simulink model "NeuronalNetwork"  (R2019b)
settings: Solver=VariableStepAuto  StartTime=0.0  StopTime=10.0  RelTol=1e-3
libraries: neural x1006
(part 1 of 11)
settings Model: Creator=Laura  LastModifiedBy=Laura

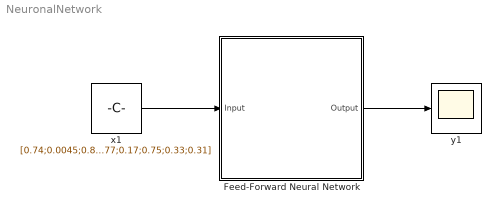
== system NeuronalNetwork ==
  Feed-Forward Neural Network : Subsystem
      mask help: Feed-Forward Neural Network
      mask Display: e = 0.06;c1 = [120 150 230]/255;c2 = ([120 150 230]+0)/383;c3 = ([120 150 230]+128)/383;patch([0 1 1 0],[0 0 1 1],c1);patch([0 1 1 1-e 1-e 0+e],[0 0 1 1-e 0+e 0+e],c2);patch([0 0 1 1-e 0+e 0+e],[0 1 1 1-e 1-e 0+e],c3);plot([0 1 1 0 0],[0 0 1 1 0]);fprintf('NNET');port_label('input',1,' Input');port_label('output',1,'Output ');
  x1 : Constant  Value=[0.74;0.0045;0.85;0.7;0.56;0.34;0.33;0.077;0.46;0.66;0.57;0.4;0.93;0.36;0.95;0.03;0.44;0.7;0.7;0.51;0.61;0.75;0.8;0.34;0.56;0.86;0.59;0.51;0.85;0.68;0.11;0.5;0.019;0.44;0.91;0.045;0.95;0.18;0.37;0.21;0.096;0.43;0.28;0.1;0.5;0.24;0.35;0.56;0.55;0.42;0.39;0.38;0.28;0.18;0.13;0.016;0.75;0.5;0.72;0.76;0.27;0.19;0.064;0.43;0.7;0.98;0.55;0.044;0.58;0.28;0.54;0.44;0.12;0.38;0.76;0.92;0.69;0.97;0.13;0.65;0.39;0.56;0.2;0.39;0.34;0.36;0.37;0.12;0.5;0.82;0.34;0.5;0.12;0.58;0.52;0.36;0.86;0.34;0.46;0.24;0.77;0.27;0.53;0.53;0.87;0.94;0.049;0.98;0.63;0.073;0.21;0.36;0.43;0.76;0.92;0.63;0.96;0.76;0.53;0.85;0.82;0.13;0.76;0.62;0.4;0.84;0.038;0.096;0.95;0.4;0.53;0.9;0.34;0.66;0.73;0.22;0.56;0.46;0.61;0.54;0.52;0.29;0.88;0.94;0.81;0.97;0.52;0.11;0.65;0.19;0.86;0.94;0.1;0.3;0.8;0.44;0.49;0.03;0.57;0.57;0.74;0.077;0.79;0.19;0.53;0.92;0.99;0.98;0.3;0.75;0.21;0.86;0.66;0.1;0.58;0.96;0.84;0.75;0.7;0.25;0.04;0.46;0.12;0.16;0.42;0.67;0.97;0.28;0.53;0.93;0.17;0.79;0.1;0.88;0.52;0.97;0.76;0.72;0.0026;0.21;0.26;0.08;0.74;0.82;0.34;0.14;0.67;0.83;0.67;0.14;0.38;0.68;0.52;0.98;0.27;0.87;0.37;0.14;0.083;0.74;0.37;0.38;0.3;0.29;0.26;0.46;0.99;0.39;0.94;0.17;0.93;0.75;0.86;0.6;0.11;0.46;0.65;0.058;0.021;0.29;0.93;0.51;0.88;0.38;0.88;0.53;0.89;0.1;0.21;0.7;0.36;0.0014;0.38;0.32;0.39;0.18;0.21;0.59;0.59;0.17;0.93;0.056;0.2;0.51;0.76;0.15;0.93;0.42;0.056;0.67;0.28;0.78;0.96;0.69;0.5;0.099;0.29;0.54;0.011;0.28;0.59;0.17;0.17;0.68;0.57;0.55;0.97;0.63;0.32;0.52;0.86;0.99;0.84;0.35;0.75;0.94;0.67;0.48;0.29;0.6;0.34;0.96;0.44;0.96;0.68;0.71;0.96;0.94;0.83;0.16;0.83;0.46;0.3;0.52;0.83;0.54;0.26;0.35;0.19;0.35;0.19;0.84;0.38;0.0095;0.31;0.84;0.28;0.78;0.53;0.15;0.53;0.28;0.71;0.73;0.45;0.18;0.14;0.27;0.64;0.81;0.67;0.29;0.14;0.25;0.69;0.072;0.5;0.99;0.9;0.58;0.77;0.75;0.7;0.68;0.28;0.58;0.62;0.81;0.016;0.21;0.99;0.82;0.63;0.68;0.81;0.28;0.66;0.029;0.54;0.53;0.87;0.19;0.93;0.98;0.33;0.62;0.53;0.46;0.36;0.33;0.083;0.39;0.24;0.49;0.7;0.14;0.83;0.93;0.83;0.48;0.66;0.46;0.42;0.034;0.93;0.043;0.48;0.39;0.53;1;0.9;0.015;0.78;0.49;0.39;0.82;0.87;1;0.2;0.87;0.31;0.41;0.82;0.37;0.43;0.091;0.67;0.73;0.3;0.34;0.73;0.99;0.7;0.09;0.47;0.64;0.53;0.14;0.28;0.99;0.79;0.93;0.35;0.21;0.68;0.36;0.44;0.91;0.83;0.39;0.73;0.29;0.29;0.3;0.025;0.92;0.69;0.23;0.5;0.79;0.38;0.22;0.72;0.77;0.69;0.62;0.76;0.51;0.33;0.0013;0.58;0.17;0.19;0.15;0.51;0.017;0.47;0.046;0.44;0.16;0.57;0.82;0.085;0.23;0.25;0.35;0.41;0.11;0.41;0.68;0.54;0.36;0.66;0.68;0.13;0.44;0.94;0.57;0.58;0.76;0.25;0.69;0.29;0.57;0.63;0.4;0.25;0.94;0.45;0.53;0.63;0.67;0.44;0.17;0.69;0.92;0.37;0.64;0.89;0.48;0.63;0.47;0.11;0.11;0.11;0.45;0.94;0.63;0.93;0.063;0.31;0.95;0.01;0.17;0.76;0.83;0.61;0.52;0.94;0.74;0.7;0.74;0.87;0.96;0.98;0.92;0.28;0.059;0.82;0.18;0.035;0.77;0.54;0.33;0.58;0.85;0.64;0.42;0.55;0.18;0.24;0.21;0.26;0.94;0.64;0.83;0.39;0.17;0.74;0.87;0.36;0.18;1;0.96;0.16;0.93;0.42;0.22;0.14;0.26;0.54;0.082;0.6;0.029;0.45;0.33;0.94;0.3;0.43;0.66;0.38;0.14;0.097;0.31;0.82;0.63;0.21;0.98;0.44;0.84;0.54;0.025;0.0068;0.79;0.45;0.29;0.86;0.66;0.28;0.64;0.26;0.17;0.37;0.54;0.93;0.75;0.15;0.0029;0.13;0.92;0.67;0.11;0.96;0.12;0.49;0.36;0.47;0.059;0.33;0.26;0.25;0.95;0.032;0.91;0.37;0.66;0.95;0.094;0.69;0.41;0.11;0.49;0.46;0.88;0.66;0.28;0.66;0.65;0.9;0.88;0.34;0.43;0.8;0.92;0.87;0.5;0.58;0.92;0.17;0.37;0.26;0.83;0.07;0.28;0.56;0.62;0.41;0.26;0.42;0.38;0.096;0.13;0.61;0.66;0.84;0.5;0.31;0.17;0.049;0.23;0.37;0.57;0.57;0.78;0.59;0.11;0.64;0.072;0.37;0.29;0.74;0.067;0.76;0.24;0.23;0.012;0.13;0.21;0.21;0.91;0.28;0.097;0.78;0.67;0.61;0.34;0.69;0.23;0.31;0.36;0.22;0.68;0.74;0.01;0.36;0.24;0.93;0.76;0.38;0.69;0.7;0.59;0.96;0.78;0.54;0.094;0.89;0.26;0.46;0.33;0.76;0.8;0.8;0.88;0.087;0.67;0.5;0.34;0.59;0.35;0.21;0.26;0.099;0.15;0.32;0.59;0.15;0.063;0.0078;0.77;0.68;0.12;0.72;0.16;0.12;0.68;0.14;0.058;0.13;0.015;0.19;0.071;0.038;0.31;0.52;0.39;1;0.44;0.15;0.78;0.74;0.088;0.47;0.29;0.41;0.43;0.87;0.71;0.014;0.025;0.24;0.6;0.93;0.33;0.44;0.099;0.72;0.72;0.78;0.94;0.048;0.8;0.47;0.28;0.045;0.79;0.9;0.78;0.84;0.34;0.19;0.38;0.26;0.021;0.29;0.24;0.2;0.35 ...(+1021 chars)]  SampleTime=0.1
      mask Display: e = 0.06;c1 = [120 230 180]/255;c2 = ([120 230 180]+0)/(256+128);c3 = ([120 230 180]+128)/(256+128);patch([0 1 1 0],[0 0 1 1],c1);patch([0 1 1 1-e 1-e 0+e],[0 0 1 1-e 0+e 0+e],c2);patch([0 0 1 1-e 0+e 0+e],[0 1 1 1-e 1-e 0+e],c3);plot([0 1 1 0 0],[0 0 1 1 0]);disp('Constant');
  y1 : Scope
      mask Display: e = 0.06;c1 = [120 230 180]/255;c2 = ([120 230 180]+0)/(256+128);c3 = ([120 230 180]+128)/(256+128);patch([0 1 1 0],[0 0 1 1],c1);patch([0 1 1 1-e 1-e 0+e],[0 0 1 1-e 0+e 0+e],c2);patch([0 0 1 1-e 0+e 0+e],[0 1 1 1-e 1-e 0+e],c3);plot([0 1 1 0 0],[0 0 1 1 0]);plot([0.15 0.85 0.85 0.15 0.15],[0.5 0.5 0.85 0.85 0.5]);
  wires:
  x1/1 -> Feed-Forward Neural Network/1(Input)
  Feed-Forward Neural Network/1(Output) -> y1/1

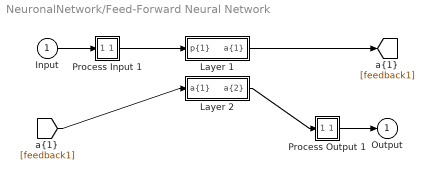
== system NeuronalNetwork/Feed-Forward Neural Network ==
  Input : Inport  PortDimensions=1001  SampleTime=0.1
      mask Display: e = 0.06;c1 = [120 230 180]/255;c2 = ([120 230 180]+0)/(256+128);c3 = ([120 230 180]+128)/(256+128);patch([0 1 1 0],[0 0 1 1],c1);patch([0 1 1 1-e 1-e 0+e],[0 0 1 1-e 0+e 0+e],c2);patch([0 0 1 1-e 0+e 0+e],[0 1 1 1-e 1-e 0+e],c3);plot([0 1 1 0 0],[0 0 1 1 0]);
  Layer 1 : Subsystem
      mask Display: e = 0.06;c1 = [120 150 230]/255;c2 = ([120 150 230]+0)/383;c3 = ([120 150 230]+128)/383;patch([0 1 1 0],[0 0 1 1],c1);patch([0 1 1 1-e 1-e 0+e],[0 0 1 1-e 0+e 0+e],c2);patch([0 0 1 1-e 0+e 0+e],[0 1 1 1-e 1-e 0+e],c3);plot([0 1 1 0 0],[0 0 1 1 0]);
  Layer 2 : Subsystem
      mask Display: e = 0.06;c1 = [120 150 230]/255;c2 = ([120 150 230]+0)/383;c3 = ([120 150 230]+128)/383;patch([0 1 1 0],[0 0 1 1],c1);patch([0 1 1 1-e 1-e 0+e],[0 0 1 1-e 0+e 0+e],c2);patch([0 0 1 1-e 0+e 0+e],[0 1 1 1-e 1-e 0+e],c3);plot([0 1 1 0 0],[0 0 1 1 0]);
  Process Input 1 : Subsystem
      mask Display: e = 0.06;c1 = [120 150 230]/255;c2 = ([120 150 230]+0)/383;c3 = ([120 150 230]+128)/383;patch([0 1 1 0],[0 0 1 1],c1);patch([0 1 1 1-e 1-e 0+e],[0 0 1 1-e 0+e 0+e],c2);patch([0 0 1 1-e 0+e 0+e],[0 1 1 1-e 1-e 0+e],c3);plot([0 1 1 0 0],[0 0 1 1 0]);
  Process Output 1 : Subsystem
      mask Display: e = 0.06;c1 = [120 150 230]/255;c2 = ([120 150 230]+0)/383;c3 = ([120 150 230]+128)/383;patch([0 1 1 0],[0 0 1 1],c1);patch([0 1 1 1-e 1-e 0+e],[0 0 1 1-e 0+e 0+e],c2);patch([0 0 1 1-e 0+e 0+e],[0 1 1 1-e 1-e 0+e],c3);plot([0 1 1 0 0],[0 0 1 1 0]);
  Output : Outport  InitialOutput=[0;0;0;0;0;0;0;0;0;0;0;0;0;0;0;0;0;0;0;0;0;0;0;0;0;0;0;0;0;0;0;0;0;0;0;0;0;0;0;0;0;0;0;0;0;0;0;0;0;0;0;0;0;0;0;0;0;0;0;0;0;0;0;0;0;0;0;0;0;0;0;0;0;0;0;0;0;0;0;0;0;0;0;0;0;0;0;0;0;0;0;0;0;0;0;0;0;0;0;0;0;0;0;0;0;0;0;0;0;0;0;0;0;0;0;0;0;0;0;0;0;0;0;0;0;0;0;0;0;0;0;0;0;0;0;0;0;0;0;0;0;0;0;0;0;0;0;0;0;0;0;0;0;0;0;0;0;0;0;0;0;0;0;0;0;0;0;0;0;0;0;0;0;0;0;0;0;0;0;0;0;0;0;0;0;0;0;0;0;0;0;0;0;0;0;0;0;0;0;0;0;0;0;0;0;0;0;0;0;0;0;0;0;0;0;0;0;0;0;0;0;0;0;0;0;0;0;0;0;0;0;0;0;0;0;0;0;0;0;0;0;0;0;0;0;0;0;0;0;0;0;0;0;0;0;0;0;0;0;0;0;0;0;0;0;0;0;0;0;0;0;0;0;0;0;0;0;0;0;0;0;0;0;0;0;0;0;0;0;0;0;0;0;0;0;0;0;0;0;0;0;0;0;0;0;0;0;0;0;0;0;0;0;0;0;0;0;0;0;0;0;0;0;0;0;0;0;0;0;0;0;0;0;0;0;0;0;0;0;0;0;0;0;0;0;0;0;0;0;0;0;0;0;0;0;0;0;0;0;0;0;0;0;0;0;0;0;0;0;0;0;0;0;0;0;0;0;0;0;0;0;0;0;0;0;0;0;0;0;0;0;0;0;0;0;0;0;0;0;0;0;0;0;0;0;0;0;0;0;0;0;0;0;0;0;0;0;0;0;0;0;0;0;0;0;0;0;0;0;0;0;0;0;0;0;0;0;0;0;0;0;0;0;0;0;0;0;0;0;0;0;0;0;0;0;0;0;0;0;0;0;0;0;0;0;0;0;0;0;0;0;0;0;0;0;0;0;0;0;0;0;0;0;0;0;0;0;0;0;0;0;0;0;0;0;0;0;0;0;0;0;0;0;0;0;0;0;0;0;0;0;0;0;0;0;0;0;0;0;0;0;0;0;0;0;0;0;0;0;0;0;0;0;0;0;0;0;0;0;0;0;0;0;0;0;0;0;0;0;0;0;0;0;0;0;0;0;0;0;0;0;0;0;0;0;0;0;0;0;0;0;0;0;0;0;0;0;0;0;0;0;0;0;0;0;0;0;0;0;0;0;0;0;0;0;0;0;0;0;0;0;0;0;0;0;0;0;0;0;0;0;0;0;0;0;0;0;0;0;0;0;0;0;0;0;0;0;0;0;0;0;0;0;0;0;0;0;0;0;0;0;0;0;0;0;0;0;0;0;0;0;0;0;0;0;0;0;0;0;0;0;0;0;0;0;0;0;0;0;0;0;0;0;0;0;0;0;0;0;0;0;0;0;0;0;0;0;0;0;0;0;0;0;0;0;0;0;0;0;0;0;0;0;0;0;0;0;0;0;0;0;0;0;0;0;0;0;0;0;0;0;0;0;0;0;0;0;0;0;0;0;0;0;0;0;0;0;0;0;0;0;0;0;0;0;0;0;0;0;0;0;0;0;0;0;0;0;0;0;0;0;0;0;0;0;0;0;0;0;0;0;0;0;0;0;0;0;0;0;0;0;0;0;0;0;0;0;0;0;0;0;0;0;0;0;0;0;0;0;0;0;0;0;0;0;0;0;0;0;0;0;0;0;0;0;0;0;0;0;0;0;0;0;0;0;0;0;0;0;0;0;0;0;0;0;0;0;0;0;0;0;0;0;0;0;0;0;0;0;0;0;0;0;0;0;0;0;0;0;0;0;0;0;0;0;0;0;0;0;0;0;0;0;0;0;0;0;0;0;0;0;0;0;0;0;0;0;0;0;0;0;0;0;0;0;0;0;0;0;0;0;0;0;0;0;0;0;0;0;0;0;0;0;0;0;0;0;0;0;0;0;0;0;0;0;0;0;0;0;0;0;0;0;0;0;0;0;0;0;0;0;0;0;0;0;0;0;0;0;0;0;0;0;0;0;0;0;0;0;0;0;0;0;0;0;0;0;0;0;0;0;0;0;0;0;0;0;0;0;0;0;0;0;0;0;0;0;0;0;0;0;0;0;0;0;0;0;0;0;0;0]
      mask Display: e = 0.06;c1 = [120 230 180]/255;c2 = ([120 230 180]+0)/(256+128);c3 = ([120 230 180]+128)/(256+128);patch([0 1 1 0],[0 0 1 1],c1);patch([0 1 1 1-e 1-e 0+e],[0 0 1 1-e 0+e 0+e],c2);patch([0 0 1 1-e 0+e 0+e],[0 1 1 1-e 1-e 0+e],c3);plot([0 1 1 0 0],[0 0 1 1 0]);
  wires:
  Input/1 -> Process Input 1/1(x)
  Process Output 1/1(y) -> Output/1
  Process Input 1/1(p) -> Layer 1/1("p{1}")
  Layer 1/1("a{1}") -> [feedback1]
  [feedback1] -> Layer 2/1("a{1} ")
  Layer 2/1("a{2}") -> Process Output 1/1(a)

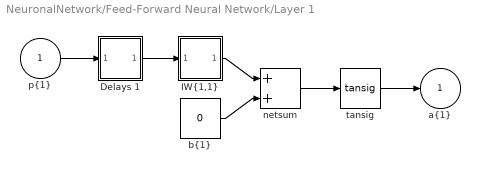
== system NeuronalNetwork/Feed-Forward Neural Network/Layer 1 ==
  "p{1}" : Inport  PortDimensions=1001  SampleTime=0.1
      mask Display: e = 0.06;c1 = [120 230 180]/255;c2 = ([120 230 180]+0)/(256+128);c3 = ([120 230 180]+128)/(256+128);patch([0 1 1 0],[0 0 1 1],c1);patch([0 1 1 1-e 1-e 0+e],[0 0 1 1-e 0+e 0+e],c2);patch([0 0 1 1-e 0+e 0+e],[0 1 1 1-e 1-e 0+e],c3);plot([0 1 1 0 0],[0 0 1 1 0]);
  Delays 1 : Subsystem
      mask Display: e = 0.06;c1 = [120 150 230]/255;c2 = ([120 150 230]+0)/383;c3 = ([120 150 230]+128)/383;patch([0 1 1 0],[0 0 1 1],c1);patch([0 1 1 1-e 1-e 0+e],[0 0 1 1-e 0+e 0+e],c2);patch([0 0 1 1-e 0+e 0+e],[0 1 1 1-e 1-e 0+e],c3);plot([0 1 1 0 0],[0 0 1 1 0]);disp('0');
  "IW{1,1}" : Subsystem
      mask Display: e = 0.06;c1 = [120 150 230]/255;c2 = ([120 150 230]+0)/383;c3 = ([120 150 230]+128)/383;patch([0 1 1 0],[0 0 1 1],c1);patch([0 1 1 1-e 1-e 0+e],[0 0 1 1-e 0+e 0+e],c2);patch([0 0 1 1-e 0+e 0+e],[0 1 1 1-e 1-e 0+e],c3);plot([0 1 1 0 0],[0 0 1 1 0]);disp('W');
  "b{1}" : Constant  Value=0
      mask Display: e = 0.06;c1 = [120 150 230]/255;c2 = ([120 150 230]+0)/383;c3 = ([120 150 230]+128)/383;patch([0 1 1 0],[0 0 1 1],c1);patch([0 1 1 1-e 1-e 0+e],[0 0 1 1-e 0+e 0+e],c2);patch([0 0 1 1-e 0+e 0+e],[0 1 1 1-e 1-e 0+e],c3);plot([0 1 1 0 0],[0 0 1 1 0]);disp('b');
  netsum : Sum  Inputs=2  SaturateOnIntegerOverflow=on  InputSameDT=on  OutDataTypeStr=Inherit: Same as first input
      mask Display: e = 0.06;c1 = [120 150 230]/255;c2 = ([120 150 230]+0)/383;c3 = ([120 150 230]+128)/383;patch([0 1 1 0],[0 0 1 1],c1);patch([0 1 1 1-e 1-e 0+e],[0 0 1 1-e 0+e 0+e],c2);patch([0 0 1 1-e 0+e 0+e],[0 1 1 1-e 1-e 0+e],c3);plot([0 1 1 0 0],[0 0 1 1 0]);disp('+');
  tansig : neural/Transfer Functions/tansig
      settings: SourceProductName=Deep Learning Toolbox
  "a{1}" : Outport  InitialOutput=0
      mask Display: e = 0.06;c1 = [120 230 180]/255;c2 = ([120 230 180]+0)/(256+128);c3 = ([120 230 180]+128)/(256+128);patch([0 1 1 0],[0 0 1 1],c1);patch([0 1 1 1-e 1-e 0+e],[0 0 1 1-e 0+e 0+e],c2);patch([0 0 1 1-e 0+e 0+e],[0 1 1 1-e 1-e 0+e],c3);plot([0 1 1 0 0],[0 0 1 1 0]);
  wires:
  "p{1}"/1 -> Delays 1/1("p{1}")
  Delays 1/1("pd{1,1}") -> "IW{1,1}"/1("pd{1,1}")
  "IW{1,1}"/1("iz{1,1}") -> netsum/1
  "b{1}"/1 -> netsum/2
  netsum/1 -> tansig/1
  tansig/1 -> "a{1}"/1
